simulink model "TC_patch"  (R2022b)
settings: Solver=FixedStepAuto  StartTime=0.0  StopTime=12  FixedStep=0.02  RelTol=1e-3
model workspace (MAT data in the model file):
  IP_SLIP_TGT = [20 3 3 4]
  IP_SLIP_TGT_X = [0 10 60 100]
  IP_SLIP_TGT_Y = [50; 100]
  TC_D = 0.01
  TC_I = 0
  TC_IGA_MAX = 0
  TC_IGA_MIN = -25
  TC_P = 1.3
libraries: slpidlib x1
settings Model: Creator=Sam  LastModifiedBy=Sam
settings RTWCC: GenCodeOnly=on

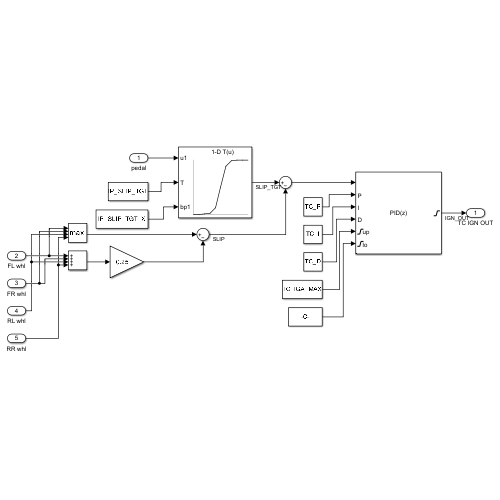
[thumbnail: Simulink's stored preview of the top-level diagram]
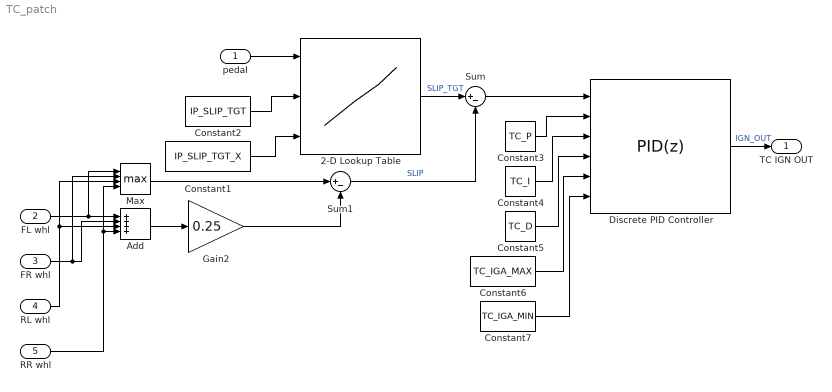
== system TC_patch ==
  pedal : Inport
  FL whl : Inport  Port=2
  FR whl : Inport  Port=3
  RL whl : Inport  Port=4
  RR whl : Inport  Port=5
  2-D Lookup Table : Lookup_n-D  NumberOfTableDimensions=1  BreakpointsForDimension1Source=Input port  BreakpointsForDimension1=[1:3]  BreakpointsForDimension2Source=Input port  BreakpointsForDimension2=[1:3]  TableSource=Input port  InterpMethod=Linear Lagrange  ExtrapMethod=Clip  UseLastTableValue=on  InternalRulePriority=Speed  RndMeth=Simplest
      settings: InputPortMap=u0,p221,p5
  Add : Sum  Inputs=++++
  Constant1 : Constant  Value=IP_SLIP_TGT_X  VectorParams1D=off
  Constant2 : Constant  Value=IP_SLIP_TGT  VectorParams1D=off
  Constant3 : Constant  Value=TC_P
  Constant4 : Constant  Value=TC_I
  Constant5 : Constant  Value=TC_D
  Constant6 : Constant  Value=TC_IGA_MAX
  Constant7 : Constant  Value=TC_IGA_MIN
  Discrete PID Controller : slpidlib/PID Controller  Controller=PID  Form=Parallel  TimeDomain=Discrete-time  UseExternalTs=off  SampleTime=-1  IntegratorMethod=Forward Euler  FilterMethod=Forward Euler  ControllerParametersSource=external  P=1  I=1  UseKiTs=off  D=0  N=100  UseFilter=off  TunerSelectOption=Transfer Function Based (PID Tuner App)  InitialConditionSource=internal  InitialConditionForIntegrator=0  InitialConditionForFilter=0  DifferentiatorICPrevScaledInput=0  ExternalReset=none  TrackingMode=off  Kt=1  LimitOutput=on  SatLimitsSource=external  UpperSaturationLimit=inf  LowerSaturationLimit=-inf  LinearizeAsGain=off  AntiWindupMode=clamping  Kb=1  LimitIntegrator=on  UpperIntegratorSaturationLimit=0  LowerIntegratorSaturationLimit=-10  POutMin=[]  POutMax=[]  IOutMin=[]  IOutMax=[]  DOutMin=[]  DOutMax=[]  NOutMin=[]  NOutMax=[]  SumOutMin=[]  SumOutMax=[]  SaturationOutMin=[]  SaturationOutMax=[]  PParamMin=[]  PParamMax=[]  IParamMin=[]  IParamMax=[]  DParamMin=[]  DParamMax=[]  NParamMin=[]  NParamMax=[]  KbParamMin=[]  KbParamMax=[]  KtParamMin=[]  KtParamMax=[]  KbOutMin=[]  KbOutMax=[]  KtOutMin=[]  KtOutMax=[]  IntegratorOutMin=[]  IntegratorOutMax=[]  FilterOutMin=[]  FilterOutMax=[]  SumI1OutMin=[]  SumI1OutMax=[]  SumI2OutMin=[]  SumI2OutMax=[]  SumI3OutMin=[]  SumI3OutMax=[]  SumI4OutMin=[]  SumI4OutMax=[]  SumDOutMin=[]  SumDOutMax=[]  DifferentiatorOutMin=[]  DifferentiatorOutMax=[]  FilterDiffOutCoefMin=[]  FilterDiffOutCoefMax=[]  ReciprocalOutMin=[]  ReciprocalOutMax=[]  SumDenOutMin=[]  SumDenOutMax=[]  SumNumOutMin=[]  SumNumOutMax=[]  DivideOutMin=[]  DivideOutMax=[]  UdiffTsProdOutMin=[]  UdiffTsProdOutMax=[]  NTsProdOutMin=[]  NTsProdOutMax=[]  UintegralTsProdOutMin=[]  UintegralTsProdOutMax=[]  UngainTsProdOutMin=[]  UngainTsProdOutMax=[]  ClampingZeroOutDataTypeStr=Inherit: Inherit via back propagation  ClampingZeroOutMin=[]  ClampingZeroOutMax=[]  FilterDenConstantOutDataTypeStr=Inherit: Inherit via back propagation  FilterDenConstantOutMin=[]  FilterDenConstantOutMax=[]  PCopyOutDataTypeStr=Inherit: Inherit via back propagation  PCopyOutMin=[]  PCopyOutMax=[]  NCopyOutDataTypeStr=Inherit: Inherit via back propagation  NCopyOutMin=[]  NCopyOutMax=[]  IntegratorContinuousStateAttributes=''  IntegratorStateMustResolveToSignalObject=off  IntegratorRTWStateStorageClass=Auto  FilterContinuousStateAttributes=''  FilterStateMustResolveToSignalObject=off  FilterRTWStateStorageClass=Auto  ParallelPVariant=ExternalParameters  IdealPVariant=Disabled  IVariant=ExternalParameters  DVariant=ExternalParameters  IntegratorVariant=Discrete  SatVariant=External  AWVariant=DiscClampingParallel  PCopyVariant=Disabled  TRVariant=Disabled  FdbkBlocksVariant=Forward  IdealPFdbkVariant=Disabled  SatFdbkVariant=Disabled  DerivativeFilterVariant=Differentiator  NVariant=Passthrough  NCopyVariant=Disabled_SignalSpec  FilterICVariant=InternalICsDifferentiator  IntegratorICVariant=InternalICs  ExternalResetVariant=Disabled  TRSumVariant=Passthrough  SumFdbkVariant=Disabled  SumVariant=Sum_PID  TsampFilterVariant=InternalTs  TsampNgainVariant=Passthrough  TsampIntegralVariant=Passthrough  ExternalSaturationOutDataTypeStr=Inherit: Same as second input
      settings: LibrarySourceBlock=simulink/Discrete/Discrete PID Controller
  Gain2 : Gain  Gain=0.25
  Max : MinMax  Function=max  Inputs=4
  Sum : Sum  Inputs=|+-
  Sum1 : Sum  Inputs=|+-
  TC IGN OUT : Outport
  wires:
  Constant4/1 -> Discrete PID Controller/3
  FL whl/1 -> Max/1, Add/1
  Add/1 -> Gain2/1
  Constant5/1 -> Discrete PID Controller/4
  FR whl/1 -> Add/2, Max/2
  Constant2/1 -> 2-D Lookup Table/2
  Sum/1 -> Discrete PID Controller/1
  RL whl/1 -> Add/3, Max/3
  RR whl/1 -> Max/4, Add/4
  Max/1 -> Sum1/1
  Gain2/1 -> Sum1/2
  pedal/1 -> 2-D Lookup Table/1
  Constant1/1 -> 2-D Lookup Table/3
  2-D Lookup Table/1 -> Sum/1  "SLIP_TGT"
  Sum1/1 -> Sum/2  "SLIP"
  Constant3/1 -> Discrete PID Controller/2
  Constant6/1 -> Discrete PID Controller/5
  Constant7/1 -> Discrete PID Controller/6
  Discrete PID Controller/1 -> TC IGN OUT/1  "IGN_OUT"
